simulink model "Controller_Designation_Simul"  (R2025a)
settings: Solver=ode4  StartTime=Tstart  StopTime=Tend  FixedStep=Tsim  RelTol=1e-3
values from neighbouring files (symbols this model uses):
  Gm_den = [1 31.1403]    [Controller_Designation_Design.m]    (also in Controller_Designation_Pole_Placement.m; Controller_Designation_Simulation.m = [1 1/tau_m])
  Gm_num = [10.88]    [Controller_Designation_Design.m]    (also in Controller_Designation_Pole_Placement.m; Controller_Designation_Simulation.m = [Km/tau_m])
  K1 = Kp / Kd    [Controller_Designation_Design.m]    (also in Controller_Designation_Pole_Placement.m; Controller_Designation_Simulation.m = 66.1315967612)
  K2 = Kd    [Controller_Designation_Design.m]    (also in Controller_Designation_Pole_Placement.m; Controller_Designation_Simulation.m = 0.00117352840074)
  Kg = 1/0.00067    (= 1492.53731343)    [Controller_Designation_Design.m]    (also in Controller_Designation_Pole_Placement.m; Controller_Designation_Simulation.m)
  Ts = 0.005    [Controller_Designation_Simulation.m]
settings Model: Creator=Ryuminseo  LastModifiedBy=Ryuminseo

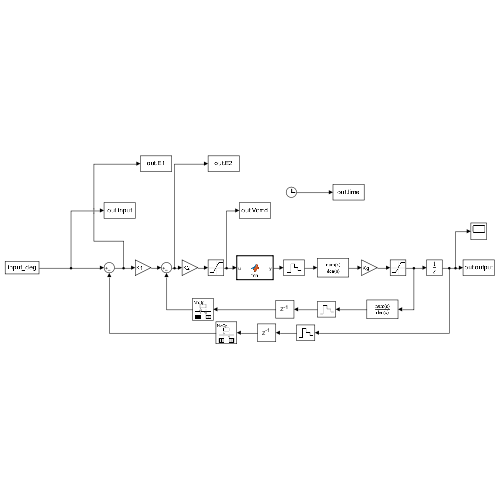
[thumbnail: Simulink's stored preview of the top-level diagram]
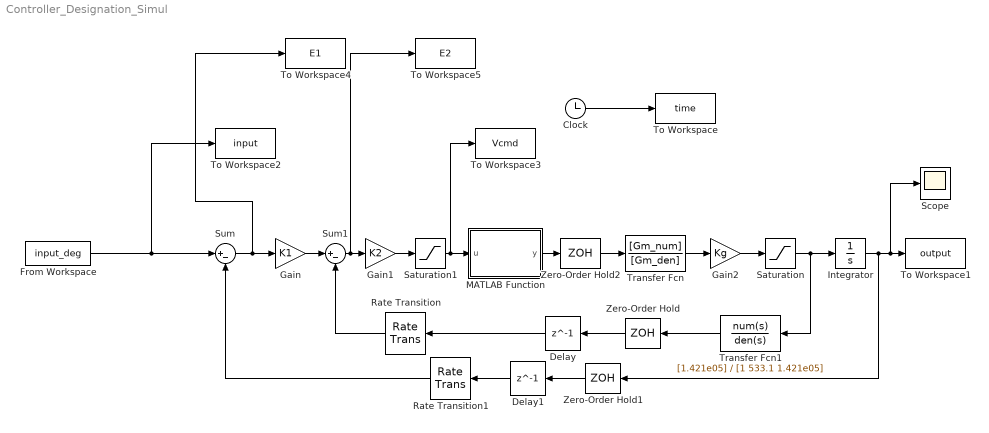
== system Controller_Designation_Simul ==
  Clock : Clock
  Delay : Delay  DelayLength=1  InitialCondition=0  SampleTime=Ts
  Delay1 : Delay  DelayLength=1  InitialCondition=0  SampleTime=Ts
  From Workspace : FromWorkspace  VariableName=input_deg  SampleTime=-1
  Gain : Gain  Gain=K1
  Gain1 : Gain  Gain=K2
  Gain2 : Gain  Gain=Kg
  Integrator : Integrator
  MATLAB Function : MATLAB Function  TreatAsAtomicUnit=on
  Rate Transition : RateTransition
  Rate Transition1 : RateTransition
  Saturation : Saturate  UpperLimit=1200  LowerLimit=-1200
  Saturation1 : Saturate  UpperLimit=2.5  LowerLimit=-2.5
  Scope : Scope
      settings: ActiveDisplayYMinimum=-1  ActiveDisplayYMaximum=1
  Sum : Sum  Inputs=|+-
  Sum1 : Sum  Inputs=|+-
  To Workspace : ToWorkspace  VariableName=time  SampleTime=-1
  To Workspace1 : ToWorkspace  VariableName=output  SampleTime=-1
  To Workspace2 : ToWorkspace  VariableName=input  SampleTime=-1
  To Workspace3 : ToWorkspace  VariableName=Vcmd  SampleTime=-1
  To Workspace4 : ToWorkspace  VariableName=E1  SampleTime=-1
  To Workspace5 : ToWorkspace  VariableName=E2  SampleTime=-1
  Transfer Fcn : TransferFcn  Numerator=[Gm_num]  Denominator=[Gm_den]
  Transfer Fcn1 : TransferFcn  Numerator=[1.421e05]  Denominator=[1 533.1 1.421e05]
  Zero-Order Hold : ZeroOrderHold  SampleTime=Ts
  Zero-Order Hold1 : ZeroOrderHold  SampleTime=Ts
  Zero-Order Hold2 : ZeroOrderHold  SampleTime=Ts
  wires:
  Transfer Fcn/1 -> Gain2/1
  Clock/1 -> To Workspace/1
  Sum/1 -> To Workspace4/1, Gain/1
  Integrator/1 -> Scope/1, To Workspace1/1, Zero-Order Hold1/1
  Delay1/1 -> Rate Transition1/1
  Delay/1 -> Rate Transition/1
  Gain1/1 -> Saturation1/1
  Gain2/1 -> Saturation/1
  Saturation/1 -> Transfer Fcn1/1, Integrator/1
  Zero-Order Hold/1 -> Delay/1
  Zero-Order Hold1/1 -> Delay1/1
  Zero-Order Hold2/1 -> Transfer Fcn/1
  Gain/1 -> Sum1/1
  Sum1/1 -> To Workspace5/1, Gain1/1
  MATLAB Function/1(y) -> Zero-Order Hold2/1
  Saturation1/1 -> To Workspace3/1, MATLAB Function/1(u)
  From Workspace/1 -> To Workspace2/1, Sum/1
  Rate Transition/1 -> Sum1/2
  Rate Transition1/1 -> Sum/2
  Transfer Fcn1/1 -> Zero-Order Hold/1

== matlab function Controller_Designation_Simul/MATLAB Function ==
  data: u input; y output
function y = fcn(u)

    if u >= -0.1 && u <= 0.1
        y = 0;
        
    else
        y = u;
    end
end
